simulink model "NMPC_model"  (Simulink 8.3)
settings: Solver=FixedStepDiscrete  StartTime=0  StopTime=Tf  FixedStep=Ts  RelTol=1e-3
values from neighbouring files (symbols this model uses):
  state = [0; 0; pi/4; 0; 0]    [robotData.m]
  Ts = 1e-3    (= 0.001)    [generate_code.m]    (also in init_sim.m)
settings Model: Creator=hirsch  LastModifiedBy=rien
settings OptimizationCC: ExpressionDepthLimit=2147483647
settings DebuggingCC: FcnCallInpInsideContextMsg=UseLocalSettings

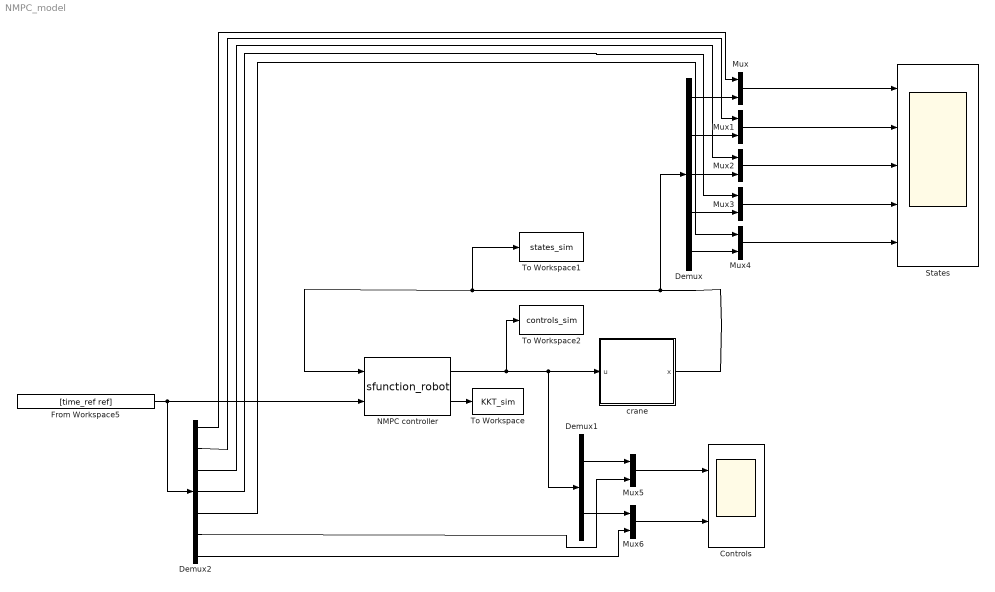
== system NMPC_model ==
  Controls : Scope  NumInputPorts=2
      settings: TimeRange=5  YMin=-5~-5  YMax=5~5
  Demux : Demux  Outputs=5
  Demux1 : Demux  Outputs=2
  Demux2 : Demux  Outputs=7
  From Workspace5 : FromWorkspace  VariableName=[time_ref ref]  SampleTime=Ts  Interpolate=off  OutputAfterFinalValue=Holding final value
  Mux{,1..6} (7 alike) : Mux  Inputs=2
  NMPC controller : S-Function  FunctionName=sfunction_robot  Parameters=Ts, xInit, uInit, S, SN, numSteps, lbV, ubV, lbAV, ubAV  EnableBusSupport=off
  States : Scope  NumInputPorts=5
      settings: TimeRange=5  YMin=-5~-5~-5~-5~-5  YMax=5~5~5~5~5
  To Workspace : ToWorkspace  VariableName=KKT_sim  SaveFormat=Structure  SampleTime=-1
  To Workspace1 : ToWorkspace  VariableName=states_sim  SaveFormat=Structure  SampleTime=-1
  To Workspace2 : ToWorkspace  VariableName=controls_sim  SaveFormat=Structure  SampleTime=-1
  crane : Subsystem
      mask help: Simple robot model. Edit <robotData.m> for configuration.
      mask init:
      | % initialize state values
      | robotData
      mask Display: disp('Robot');
  wires:
  NMPC controller/1 -> To Workspace2/1, crane/1(u), Demux1/1
  NMPC controller/2 -> To Workspace/1
  From Workspace5/1 -> NMPC controller/2, Demux2/1
  crane/1(x) -> NMPC controller/1, To Workspace1/1, Demux/1
  Demux/1 -> Mux/2
  Demux/4 -> Mux3/2
  Demux/2 -> Mux1/2
  Demux/3 -> Mux2/2
  Demux/5 -> Mux4/2
  Demux2/1 -> Mux/1
  Demux2/2 -> Mux1/1
  Demux2/3 -> Mux2/1
  Demux2/4 -> Mux3/1
  Demux2/5 -> Mux4/1
  Mux/1 -> States/1
  Mux1/1 -> States/2
  Mux2/1 -> States/3
  Mux3/1 -> States/4
  Mux4/1 -> States/5
  Demux1/1 -> Mux5/1
  Demux1/2 -> Mux6/1
  Demux2/6 -> Mux5/2
  Demux2/7 -> Mux6/2
  Mux5/1 -> Controls/1
  Mux6/1 -> Controls/2

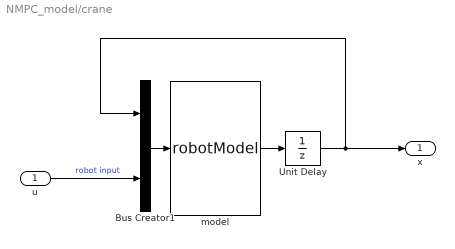
== system NMPC_model/crane ==
  u : Inport
  Bus Creator1 : BusCreator  Inputs=2
  Unit Delay : UnitDelay  InitialCondition=state  SampleTime=Ts
  model : S-Function  FunctionName=robotModel  EnableBusSupport=off
  x : Outport
  wires:
  u/1 -> Bus Creator1/2  "robot input"
  Bus Creator1/1 -> model/1
  model/1 -> Unit Delay/1
  Unit Delay/1 -> Bus Creator1/1, x/1
